simulink model "subsystem_practice"  (R2014a)
settings: Solver=ode45  StartTime=0.0  StopTime=100  RelTol=1e-3
settings Model: Creator=Huanglei  LastModifiedBy=Huanglei

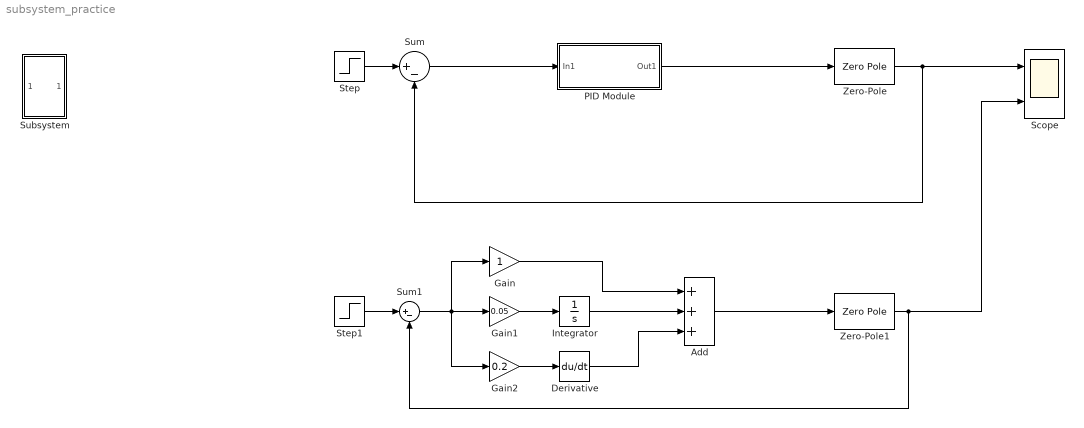
== system subsystem_practice ==
  Add : Sum  Inputs=+++
  Derivative : Derivative
  Gain : Gain
  Gain1 : Gain  Gain=0.05
  Gain2 : Gain  Gain=0.2
  Integrator : Integrator
  PID Module : Subsystem
  Scope : Scope  NumInputPorts=2
      settings: YMin=-5~-5  YMax=5~5
  Step : Step  SampleTime=0
  Step1 : Step  SampleTime=0
  Subsystem : Subsystem  mask(PID controller){Kp=1, Ki=0.05, Kd=0.2, sat_upper=10, sat_lower=-10}
      mask prompts: Kp "Parameter_Kp"; Ki "Parameter_Ki"; Kd "Parameter_Kd"; sat_upper "Saturation_up"; sat_lower "Saturation_low"
      mask help: A PID controller with saturation
      mask Help: MATLAB subsystem
  Sum : Sum  Inputs=|+-
  Sum1 : Sum  Inputs=|+-
  Zero-Pole : ZeroPole  Zeros=[]  Poles=[0 -0.5]
  Zero-Pole1 : ZeroPole  Zeros=[]  Poles=[0 -0.5]
  wires:
  Step/1 -> Sum/1
  Zero-Pole/1 -> Sum/2, Scope/1
  Step1/1 -> Sum1/1
  Sum1/1 -> Gain2/1, Gain/1, Gain1/1
  Gain1/1 -> Integrator/1
  Gain2/1 -> Derivative/1
  Gain/1 -> Add/1
  Integrator/1 -> Add/2
  Derivative/1 -> Add/3
  Add/1 -> Zero-Pole1/1
  Zero-Pole1/1 -> Scope/2, Sum1/2
  Sum/1 -> PID Module/1(In1)
  PID Module/1(Out1) -> Zero-Pole/1

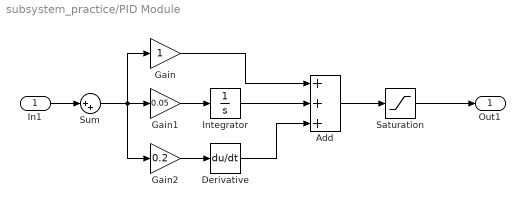
== system subsystem_practice/PID Module ==
  In1 : Inport
  Add : Sum  Inputs=+++
  Derivative : Derivative
  Gain : Gain
  Gain1 : Gain  Gain=0.05
  Gain2 : Gain  Gain=0.2
  Integrator : Integrator
  Saturation : Saturate  UpperLimit=10  LowerLimit=-10
  Sum : Sum  Inputs=|++
  Out1 : Outport
  wires:
  Sum/1 -> Gain2/1, Gain/1, Gain1/1
  Gain1/1 -> Integrator/1
  Gain2/1 -> Derivative/1
  Gain/1 -> Add/1
  Derivative/1 -> Add/3
  Integrator/1 -> Add/2
  Add/1 -> Saturation/1
  In1/1 -> Sum/1
  Saturation/1 -> Out1/1

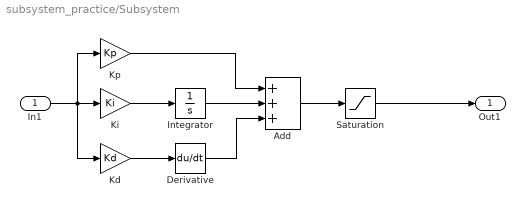
== system subsystem_practice/Subsystem ==
  In1 : Inport
  Add : Sum  Inputs=+++
  Derivative : Derivative
  Integrator : Integrator
  Kd : Gain  Gain=Kd
  Ki : Gain  Gain=Ki
  Kp : Gain  Gain=Kp
  Saturation : Saturate  UpperLimit=sat_upper  LowerLimit=sat_lower
  Out1 : Outport
  wires:
  In1/1 -> Kd/1, Kp/1, Ki/1
  Kd/1 -> Derivative/1
  Add/1 -> Saturation/1
  Ki/1 -> Integrator/1
  Integrator/1 -> Add/2
  Kp/1 -> Add/1
  Derivative/1 -> Add/3
  Saturation/1 -> Out1/1
